simulink model "V5_Modell_DCDC"  (R2022b)
settings: Solver=ode3  StartTime=0.0  StopTime=Zeit(end)  FixedStep=1e-6  RelTol=1e-3
settings Model: Creator=JSCHB  LastModifiedBy=Patrick

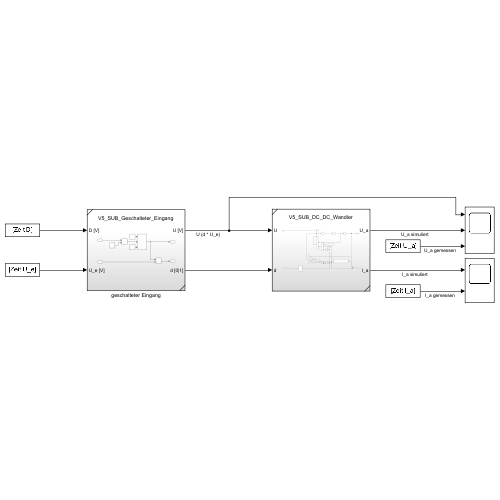
[thumbnail: Simulink's stored preview of the top-level diagram]
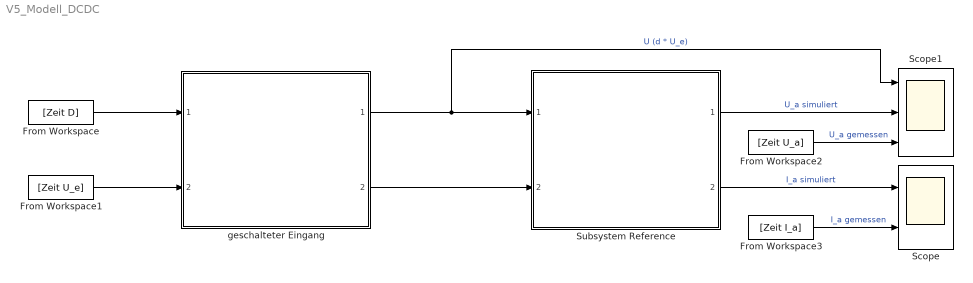
== system V5_Modell_DCDC ==
  From Workspace : FromWorkspace  VariableName=[Zeit D]
  From Workspace1 : FromWorkspace  VariableName=[Zeit U_e]
  From Workspace2 : FromWorkspace  VariableName=[Zeit U_a]
  From Workspace3 : FromWorkspace  VariableName=[Zeit I_a]
  Scope : Scope  NumInputPorts=2
  Scope1 : Scope  NumInputPorts=3
  Subsystem Reference : Subsystem  ReferencedSubsystem=V5_SUB_DC_DC_Wandler
  geschalteter Eingang : Subsystem  ReferencedSubsystem=V5_SUB_Geschalteter_Eingang
  wires:
  geschalteter Eingang/1 -> Scope1/1, Subsystem Reference/1  "U (d * U_e)"
  geschalteter Eingang/2 -> Subsystem Reference/2
  From Workspace1/1 -> geschalteter Eingang/2
  From Workspace/1 -> geschalteter Eingang/1
  Subsystem Reference/1 -> Scope1/2  "U_a simuliert"
  From Workspace2/1 -> Scope1/3  "U_a gemessen"
  From Workspace3/1 -> Scope/2  "I_a gemessen"
  Subsystem Reference/2 -> Scope/1  "I_a simuliert"
